simulink model "sampleModel1711"  (R2023a)
settings: Solver=VariableStepAuto  StartTime=0.0  StopTime=10.0  RelTol=1e-3
libraries: hdlsllib x3, simulink x1
settings Model: Creator=user1  LastModifiedBy=user1

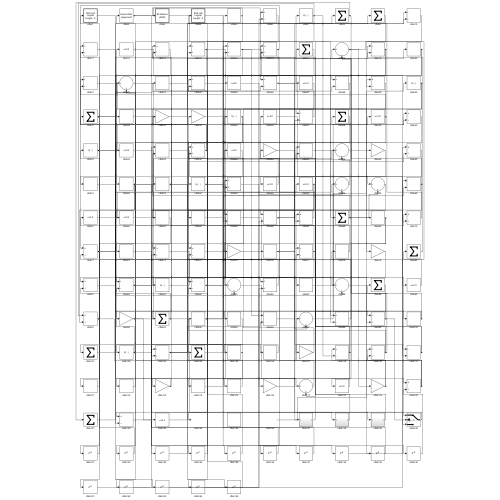
[thumbnail: Simulink's stored preview of the top-level diagram]
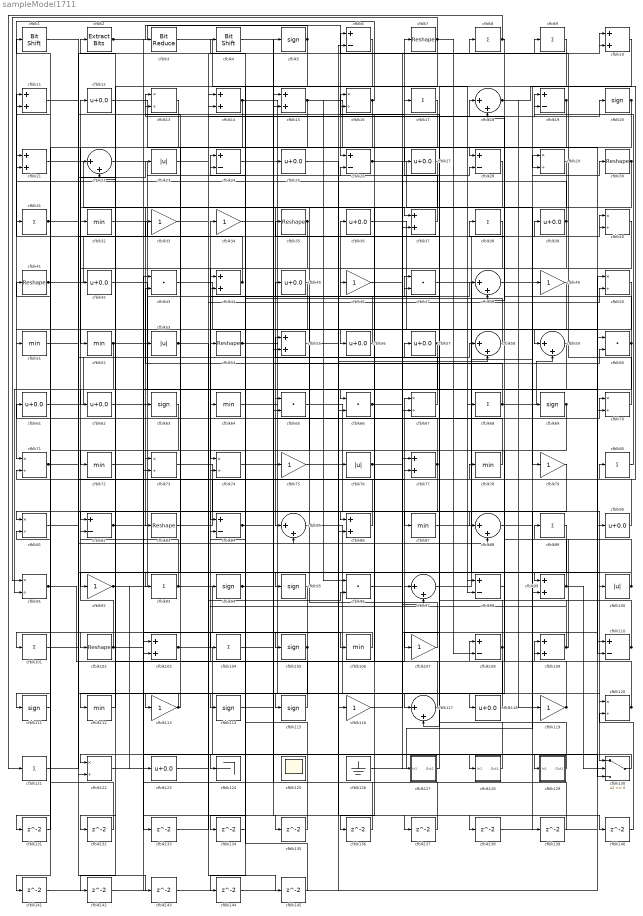
== system sampleModel1711 ==
  cfblk1 : hdlsllib/Logic and Bit Operations/Bit Shift  mode=Shift Left Logical  N=0
  cfblk{10..11,14..15,21,37,44,55,77,86,99,103,109} (13 alike) : Sum
  cfblk{23,53,76,100} (4 alike) : Abs  SaturateOnIntegerOverflow=off
  cfblk{8..9,17,31,38,68,80,89,93,101,104,121} (12 alike) : Sum  Inputs=+
  cfblk{7,30,35,41,54,83,102} (7 alike) : Reshape
  cfblk{5,20,63,69,94..95,105,111,114..115} (10 alike) : Signum
  cfblk{32,51..52,64,72,78,87,106,112} (9 alike) : MinMax
  cfblk{33..34,46,49,75,79,92,107,113,116,119} (11 alike) : Gain
  cfblk{6,19,24,26,28,82,84,98,108,110} (10 alike) : Sum  Inputs=+-
  cfblk{18,22,48,58..59,85,88,97,117} (9 alike) : Sum  Inputs=|++
  cfblk{12,25,27,36,39,42,45,56..57,61..62,90,118,123} (14 alike) : Bias  Bias=0.0  SaturateOnIntegerOverflow=off
  cfblk{13,16,29,40,50,67,70..71,73..74,81,91,120,122} (14 alike) : Product  Inputs=*/  RndMeth=Zero  SaturateOnIntegerOverflow=on
  cfblk124 : Terminator
  cfblk125 : Scope
      settings: Floating=on
  cfblk126 : Ground
  cfblk127 : Subsystem
      settings: LibrarySourceBlock=|
      | hdlsllib/Ports &
      | Subsystems/Subsystem
  cfblk128 : Subsystem
      settings: LibrarySourceBlock=|
      | hdlsllib/Ports &
      | Subsystems/Subsystem
  cfblk129 : Subsystem
      settings: LibrarySourceBlock=|
      | hdlsllib/Ports &
      | Subsystems/Subsystem
  cfblk130 : Switch  SaturateOnIntegerOverflow=off  InputSameDT=off
  cfblk{131..145} (15 alike) : Delay  SampleTime=1
  cfblk2 : simulink/Logic and Bit Operations/Extract Bits  bitsToExtract=Upper half  numBits=8  bitIdxRange=[0 7]  outScalingMode=Preserve fixed-point scaling
      settings: LibrarySourceBlock=|
      | hdlsllib/Logic and Bit
      | Operations/Extract Bits
  cfblk3 : hdlsllib/Logic and Bit Operations/Bit Reduce  mode=AND
  cfblk4 : hdlsllib/Logic and Bit Operations/Bit Shift  mode=Shift Left Logical  N=0
  cfblk{43,47,60,65..66,96} (6 alike) : DotProduct  OutDataTypeStr=Inherit: Inherit via internal rule
  wires:
  cfblk102/1 -> cfblk12/1, cfblk106/1
  cfblk5/1 -> cfblk72/1, cfblk3/1
  cfblk130/1 -> cfblk122/1
  cfblk91/1 -> cfblk67/1, cfblk31/1
  cfblk21/1 -> cfblk37/1
  cfblk115/1 -> cfblk34/1
  cfblk31/1 -> cfblk17/1, cfblk143/1
  cfblk13/1 -> cfblk52/1
  cfblk80/1 -> cfblk19/1
  cfblk2/1 -> cfblk26/1, cfblk128/1(In1)
  cfblk36/1 -> cfblk59/1
  cfblk16/1 -> cfblk71/1, cfblk114/1
  cfblk14/1 -> cfblk117/1, cfblk73/1
  cfblk89/1 -> cfblk117/2
  cfblk119/1 -> cfblk2/1, cfblk78/1
  cfblk56/1 -> cfblk36/1
  cfblk127/1(Out1) -> cfblk47/1
  cfblk44/1 -> cfblk11/1, cfblk21/1
  cfblk18/1 -> cfblk80/1, cfblk119/1
  cfblk121/1 -> cfblk40/1
  cfblk47/1 -> cfblk99/1
  cfblk103/1 -> cfblk129/1(In1), cfblk50/2, cfblk96/2
  cfblk97/1 -> cfblk39/1
  cfblk29/1 -> cfblk85/1
  cfblk1/1 -> cfblk95/1
  cfblk92/1 -> cfblk58/1, cfblk123/1
  cfblk113/1 -> cfblk112/1, cfblk13/2
  cfblk26/1 -> cfblk79/1, cfblk130/3
  cfblk116/1 -> cfblk10/1
  cfblk6/1 -> cfblk124/1
  cfblk98/1 -> cfblk18/1
  cfblk79/1 -> cfblk82/1
  cfblk90/1 -> cfblk41/1
  cfblk82/1 -> cfblk87/1, cfblk138/1
  cfblk73/1 -> cfblk86/1
  cfblk30/1 -> cfblk75/1, cfblk136/1
  cfblk77/1 -> cfblk22/1, cfblk131/1
  cfblk86/1 -> cfblk24/1
  cfblk33/1 -> cfblk20/1
  cfblk27/1 -> cfblk83/1
  cfblk94/1 -> cfblk70/1, cfblk98/2
  cfblk109/1 -> cfblk89/1, cfblk61/1, cfblk94/1
  cfblk66/1 -> cfblk19/2, cfblk48/1
  cfblk52/1 -> cfblk47/2, cfblk91/2, cfblk62/1, cfblk65/1
  cfblk59/1 -> cfblk66/1
  cfblk39/1 -> cfblk74/1, cfblk21/2
  cfblk62/1 -> cfblk26/2
  cfblk110/1 -> cfblk38/1, cfblk44/1
  cfblk118/1 -> cfblk97/1
  cfblk54/1 -> cfblk116/1, cfblk140/1
  cfblk28/1 -> cfblk32/1
  cfblk41/1 -> cfblk14/1, cfblk85/2
  cfblk38/1 -> cfblk42/1
  cfblk35/1 -> cfblk54/1, cfblk63/1
  cfblk7/1 -> cfblk91/1, cfblk65/2, cfblk108/2
  cfblk107/1 -> cfblk45/1
  cfblk32/1 -> cfblk40/2
  cfblk37/1 -> cfblk7/1
  cfblk3/1 -> cfblk98/1
  cfblk105/1 -> cfblk101/1, cfblk113/1
  cfblk65/1 -> cfblk99/2
  cfblk114/1 -> cfblk5/1
  cfblk95/1 -> cfblk102/1
  cfblk129/1(Out1) -> cfblk71/2
  cfblk112/1 -> cfblk82/2
  cfblk76/1 -> cfblk37/2, cfblk110/2
  cfblk23/1 -> cfblk9/1
  cfblk126/1 -> cfblk29/1
  cfblk20/1 -> cfblk28/1, cfblk142/1
  cfblk58/1 -> cfblk4/1
  cfblk123/1 -> cfblk8/1
  cfblk128/1(Out1) -> cfblk35/1
  cfblk42/1 -> cfblk70/2
  cfblk17/1 -> cfblk111/1
  cfblk74/1 -> cfblk130/1
  cfblk22/1 -> cfblk28/2
  cfblk68/1 -> cfblk59/2, cfblk53/1, cfblk69/1
  cfblk4/1 -> cfblk27/1
  cfblk43/1 -> cfblk90/1
  cfblk93/1 -> cfblk105/1, cfblk22/2
  cfblk85/1 -> cfblk127/1(In1)
  cfblk117/1 -> cfblk46/1
  cfblk81/1 -> cfblk23/1
  cfblk84/1 -> cfblk60/2, cfblk88/2
  cfblk87/1 -> cfblk30/1
  cfblk8/1 -> cfblk121/1, cfblk48/2
  cfblk64/1 -> cfblk97/2
  cfblk19/1 -> cfblk122/2, cfblk55/2
  cfblk51/1 -> cfblk88/1
  cfblk101/1 -> cfblk10/2
  cfblk34/1 -> cfblk120/1
  cfblk106/1 -> cfblk104/1
  cfblk50/1 -> cfblk56/1
  cfblk55/1 -> cfblk58/2
  cfblk25/1 -> cfblk76/1
  cfblk11/1 -> cfblk115/1
  cfblk10/1 -> cfblk107/1
  cfblk70/1 -> cfblk6/1
  cfblk104/1 -> cfblk25/1
  cfblk45/1 -> cfblk51/1
  cfblk46/1 -> cfblk77/1
  cfblk99/1 -> cfblk74/2, cfblk130/2
  cfblk24/1 -> cfblk15/2
  cfblk83/1 -> cfblk6/2
  cfblk67/1 -> cfblk16/1
  cfblk120/1 -> cfblk109/1, cfblk108/1, cfblk109/2
  cfblk71/1 -> cfblk77/2, cfblk57/1
  cfblk9/1 -> cfblk29/2
  cfblk60/1 -> cfblk103/2, cfblk18/2
  cfblk49/1 -> cfblk64/1
  cfblk15/1 -> cfblk84/1, cfblk68/1, cfblk96/1
  cfblk57/1 -> cfblk81/1, cfblk134/1
  cfblk100/1 -> cfblk13/1, cfblk92/1
  cfblk111/1 -> cfblk81/2
  cfblk12/1 -> cfblk110/1
  cfblk53/1 -> cfblk67/2, cfblk145/1
  cfblk61/1 -> cfblk43/2
  cfblk69/1 -> cfblk118/1, cfblk93/1
  cfblk96/1 -> cfblk100/1
  cfblk108/1 -> cfblk55/1, cfblk16/2, cfblk144/1
  cfblk48/1 -> cfblk49/1
  cfblk78/1 -> cfblk33/1
  cfblk131/1 -> cfblk1/1
  cfblk40/1 -> cfblk132/1
  cfblk132/1 -> cfblk11/2
  cfblk122/1 -> cfblk133/1
  cfblk133/1 -> cfblk14/2
  cfblk134/1 -> cfblk84/2
  cfblk72/1 -> cfblk135/1
  cfblk135/1 -> cfblk24/2
  cfblk136/1 -> cfblk103/1
  cfblk75/1 -> cfblk137/1
  cfblk137/1 -> cfblk15/1
  cfblk138/1 -> cfblk50/1
  cfblk88/1 -> cfblk139/1
  cfblk139/1 -> cfblk43/1
  cfblk140/1 -> cfblk120/2
  cfblk63/1 -> cfblk141/1
  cfblk141/1 -> cfblk66/2
  cfblk142/1 -> cfblk73/2
  cfblk143/1 -> cfblk60/1
  cfblk144/1 -> cfblk86/2
  cfblk145/1 -> cfblk44/2

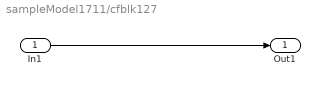
== system sampleModel1711/cfblk127 ==
  In1 : Inport
  Out1 : Outport
  wires:
  In1/1 -> Out1/1

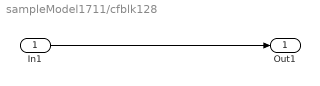
== system sampleModel1711/cfblk128 ==
  In1 : Inport
  Out1 : Outport
  wires:
  In1/1 -> Out1/1

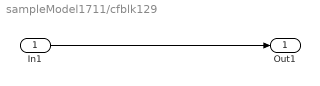
== system sampleModel1711/cfblk129 ==
  In1 : Inport
  Out1 : Outport
  wires:
  In1/1 -> Out1/1
